simulink model "RCLowPassFilter"  (R2018b)
settings: Solver=FixedStepAuto  StartTime=0.0  StopTime=10.0  FixedStep=0.01  RelTol=1e-3
settings Model: Creator=novauto  LastModifiedBy=novauto

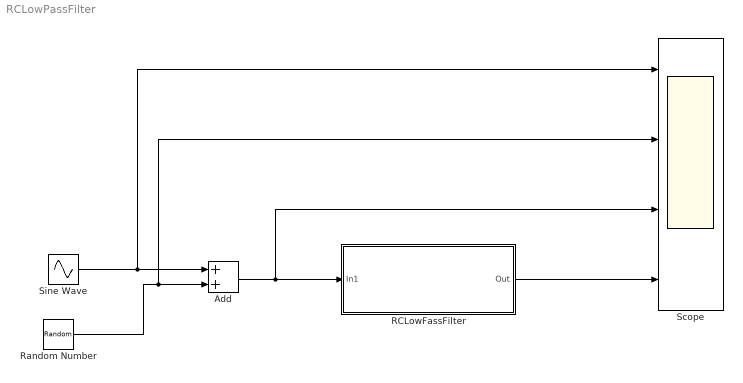
== system RCLowPassFilter ==
  Add : Sum
  RCLowFassFilter : Subsystem
  Random Number : RandomNumber
  Scope : Scope  NumInputPorts=4
  Sine Wave : Sin  Amplitude=3  SampleTime=0
  wires:
  Sine Wave/1 -> Scope/1, Add/1
  Add/1 -> Scope/3, RCLowFassFilter/1(In1)
  Random Number/1 -> Scope/2, Add/2
  RCLowFassFilter/1(Out) -> Scope/4

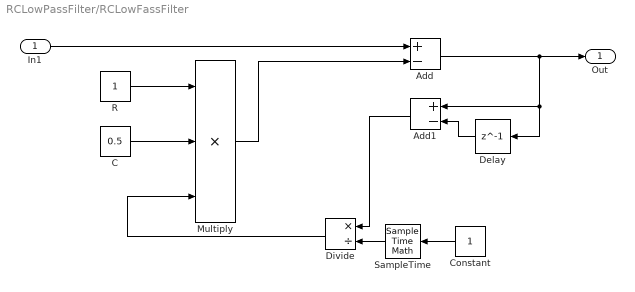
== system RCLowPassFilter/RCLowFassFilter ==
  In1 : Inport
  Add : Sum  Inputs=+-
  Add1 : Sum  Inputs=+-
  C : Constant  Value=0.5
  Constant : Constant
  Delay : Delay  DelayLength=1  InitialCondition=0
  Divide : Product  Inputs=*/
  Multiply : Product  Inputs=3
  R : Constant
  SampleTime : SampleTimeMath  TsampMathOp=Ts Only
  Out : Outport
  wires:
  R/1 -> Multiply/1
  C/1 -> Multiply/2
  In1/1 -> Add/1
  Add/1 -> Add1/1, Delay/1, Out/1
  Delay/1 -> Add1/2
  Add1/1 -> Divide/1
  Constant/1 -> SampleTime/1
  SampleTime/1 -> Divide/2
  Divide/1 -> Multiply/3
  Multiply/1 -> Add/2
